simulink model "full_controller_pid"  (R2024a)
settings: Solver=FixedStepAuto  StartTime=0.0  StopTime=50  FixedStep=sample_time  RelTol=1e-3
values from neighbouring files (symbols this model uses):
  dPOSG = [0; 0; 1]    [full_pid_loader.m]
  p_KD = -.01    (= -0.01)    [full_pid_loader.m]
  p_KI = 1    [full_pid_loader.m]
  p_KI_lim = 10*(2*pi/360)    (= 0.174532925199)    [full_pid_loader.m]
  p_KP = 2.7    [full_pid_loader.m]
  phi_KD = 0    [full_pid_loader.m]
  phi_KI = 0    [full_pid_loader.m]
  phi_KI_lim = 2*(2*pi/360)    (= 0.0349065850399)    [full_pid_loader.m]
  phi_KP = 4.5    [full_pid_loader.m]
  phi_max = pi/4    (= 0.785398163397)    [full_pid_loader.m]
  psi_KD = 0    [full_pid_loader.m]
  psi_KI = 0    [full_pid_loader.m]
  psi_KI_lim = 8*(2*pi/360)    (= 0.13962634016)    [full_pid_loader.m]
  psi_KP = 10    [full_pid_loader.m]
  PSIdes = 0    [full_pid_loader.m]
  q_KD = -.01    (= -0.01)    [full_pid_loader.m]
  q_KI = 1    [full_pid_loader.m]
  q_KI_lim = 10*(2*pi/360)    (= 0.174532925199)    [full_pid_loader.m]
  q_KP = 2.7    [full_pid_loader.m]
  r_KD = -.01    (= -0.01)    [full_pid_loader.m]
  r_KI = 1    [full_pid_loader.m]
  r_KI_lim = 10*(2*pi/360)    (= 0.174532925199)    [full_pid_loader.m]
  r_KP = 2.7    [full_pid_loader.m]
  theta_KD = 0    [full_pid_loader.m]
  theta_KI = 0    [full_pid_loader.m]
  theta_KI_lim = 2*(2*pi/360)    (= 0.0349065850399)    [full_pid_loader.m]
  theta_KP = 4.5    [full_pid_loader.m]
  theta_max = pi/4    (= 0.785398163397)    [full_pid_loader.m]
  X_KD = -.35    (= -0.35)    [full_pid_loader.m]
  X_KI = .25    (= 0.25)    [full_pid_loader.m]
  X_KI_lim = 10    [full_pid_loader.m]
  X_KP = .35    (= 0.35)    [full_pid_loader.m]
  Y_KD = -.35    (= -0.35)    [full_pid_loader.m]
  Y_KI = .25    (= 0.25)    [full_pid_loader.m]
  Y_KI_lim = .25    (= 0.25)    [full_pid_loader.m]
  Y_KP = .35    (= 0.35)    [full_pid_loader.m]
undefined symbols (not defined in the file or in its folder): drag_mat, g, J, Jr, m, U_max, U_min
settings Model: Creator=Lorenzo-Desk  LastModifiedBy=Lorenzo-Desk

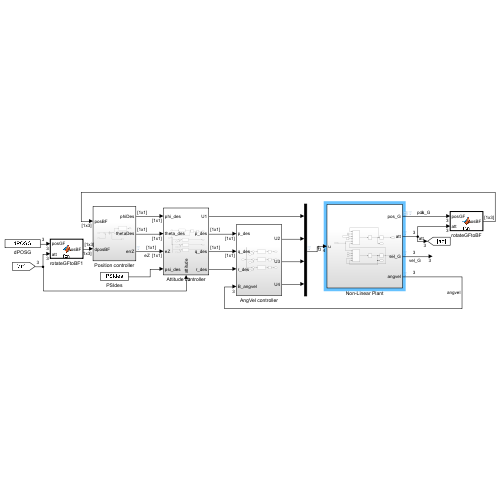
[thumbnail: Simulink's stored preview of the top-level diagram]
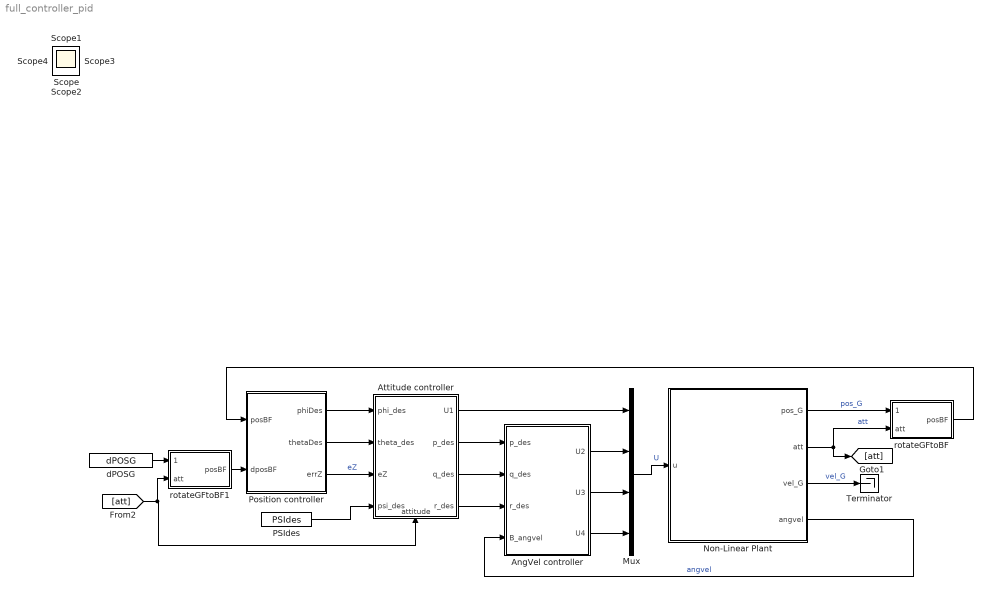
== system full_controller_pid ==
  AngVel controller : Subsystem
  Attitude controller : Subsystem
      settings: PortSchema="{\"entries\":[{\"content\":{\"sides\":[{\"content\":{\"connectorIds\":[\"In1\",\"In2\",\"In3\",\"In4\"]},\"type\":\"ConnectorPlacement.EquallySpacedRectSide\",\"uuid\":\"71281286-38ad-4f2a-91ae-9e6c4e0e30b2\"},{\"content\":{\"connectorIds\":[\"Out1\",\"Out2\",\"Out3\",\"Out4\"],\"side\":\"RIGHT\"},\"type\":\"ConnectorPlacement.EquallySpacedRectSide\",\"uuid\":\"aa649c5f-8758-4d82-8660-affbe0ed2eed\"},{\"content\":{\"side\":\"TOP\"},\"type\":\"ConnectorPlacement.EquallySpacedRectSide\",\"uuid\":\"ccfea5cf-4a16-4d49-8c61-fb0c2c5d9d69\"},{\"content\":{\"connectorIds\":[\"In5\"],\"side\":\"BOTTOM\"},\"type\":\"ConnectorPlacement.EquallySpacedRectSide\",\"uuid\":\"66e9e909-a7d3-4870-b7d3-735590f045d2\"}]},\"type\":\"ConnectorPlacement.EquallySpacedConnector\",\"uuid\":\"1ea574e8-8b7c-489a-8841-cd1e9d9d608b\"}],\"packageUris\":[\"http://schema.mathworks.com/mf0/Connector/R2020b\"],\"version\":\"1.0\"}"
  Mux : Mux
  Non-Linear Plant : Subsystem
  PSIdes : Constant  Value=PSIdes
  Position controller : Subsystem
  Terminator : Terminator
  dPOSG : Constant  Value=dPOSG
  rotateGFtoBF : MATLAB Function  TreatAsAtomicUnit=on
  rotateGFtoBF1 : MATLAB Function  TreatAsAtomicUnit=on
  Scope{,1..4} (5 alike) : Scope
  wires:
  Non-Linear Plant/1(pos_G) -> rotateGFtoBF/1(posGF)  "pos_G"
  Attitude controller/2(p_des) -> AngVel controller/1(p_des)
  PSIdes/1 -> Attitude controller/4(psi_des)
  Attitude controller/3(q_des) -> AngVel controller/2(q_des)
  Attitude controller/4(r_des) -> AngVel controller/3(r_des)
  Attitude controller/1(U1) -> Mux/1
  AngVel controller/1(U2) -> Mux/2
  AngVel controller/2(U3) -> Mux/3
  AngVel controller/3(U4) -> Mux/4
  Non-Linear Plant/2(att) -> [att], rotateGFtoBF/2(att)  "att"
  Non-Linear Plant/4(angvel) -> AngVel controller/4(B_angvel)  "angvel"
  Non-Linear Plant/3(vel_G) -> Terminator/1  "vel_G"
  Position controller/3(errZ) -> Attitude controller/3(eZ)  "eZ"
  Position controller/1(phiDes) -> Attitude controller/1(phi_des)
  Position controller/2(thetaDes) -> Attitude controller/2(theta_des)
  Mux/1 -> Non-Linear Plant/1(u)  "U"
  rotateGFtoBF/1(posBF) -> Position controller/1(posBF)
  rotateGFtoBF1/1(posBF) -> Position controller/2(dposBF)
  dPOSG/1 -> rotateGFtoBF1/1(posGF)
  [att] -> Attitude controller/5(attitude), rotateGFtoBF1/2(att)

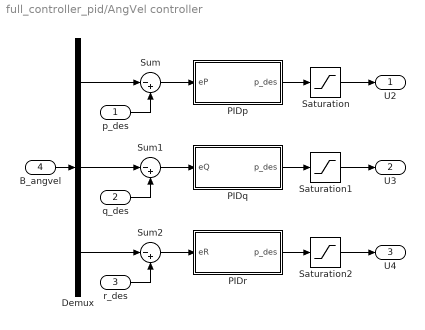
== system full_controller_pid/AngVel controller ==
  p_des : Inport
  q_des : Inport  Port=2
  r_des : Inport  Port=3
  B_angvel : Inport  Port=4
  Demux : Demux  Outputs=3
  PIDp : Subsystem
  PIDq : Subsystem
  PIDr : Subsystem
  Saturation : Saturate  UpperLimit=U_max(2)  LowerLimit=U_min(2)
  Saturation1 : Saturate  UpperLimit=U_max(3)  LowerLimit=U_min(3)
  Saturation2 : Saturate  UpperLimit=U_max(4)  LowerLimit=U_min(4)
  Sum : Sum  Inputs=|-+
  Sum1 : Sum  Inputs=|-+
  Sum2 : Sum  Inputs=|-+
  U2 : Outport
  U3 : Outport  Port=2
  U4 : Outport  Port=3
  wires:
  PIDp/1(p_des) -> Saturation/1
  PIDq/1(p_des) -> Saturation1/1
  PIDr/1(p_des) -> Saturation2/1
  Sum/1 -> PIDp/1(eP)
  Sum1/1 -> PIDq/1(eQ)
  Sum2/1 -> PIDr/1(eR)
  p_des/1 -> Sum/2
  q_des/1 -> Sum1/2
  r_des/1 -> Sum2/2
  B_angvel/1 -> Demux/1
  Demux/1 -> Sum/1
  Demux/2 -> Sum1/1
  Demux/3 -> Sum2/1
  Saturation/1 -> U2/1
  Saturation1/1 -> U3/1
  Saturation2/1 -> U4/1

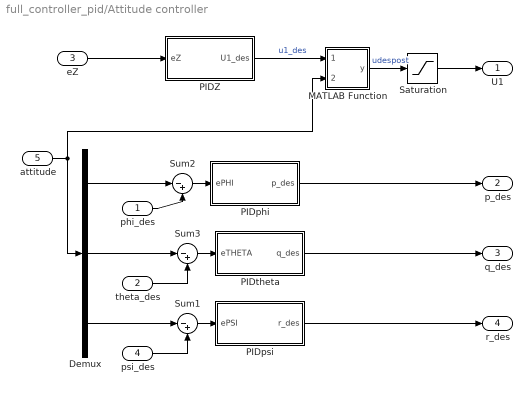
== system full_controller_pid/Attitude controller ==
  phi_des : Inport
  theta_des : Inport  Port=2
  eZ : Inport  Port=3
  psi_des : Inport  Port=4
  attitude : Inport  Port=5
  Demux : Demux  Outputs=3
  MATLAB Function : MATLAB Function  TreatAsAtomicUnit=on
  PIDZ : Subsystem
  PIDphi : Subsystem
  PIDpsi : Subsystem
  PIDtheta : Subsystem
  Saturation : Saturate  UpperLimit=U_max(1)  LowerLimit=U_min(1)
  Sum1 : Sum  Inputs=|-+
  Sum2 : Sum  Inputs=|-+
  Sum3 : Sum  Inputs=|-+
  U1 : Outport
  p_des : Outport  Port=2
  q_des : Outport  Port=3
  r_des : Outport  Port=4
  wires:
  PIDZ/1(U1_des) -> MATLAB Function/1(pidOut)  "u1_des"
  attitude/1 -> Demux/1, MATLAB Function/2(angles)
  eZ/1 -> PIDZ/1(eZ)
  PIDphi/1(p_des) -> p_des/1
  PIDtheta/1(q_des) -> q_des/1
  Sum2/1 -> PIDphi/1(ePHI)
  phi_des/1 -> Sum2/2
  Demux/1 -> Sum2/1
  Sum3/1 -> PIDtheta/1(eTHETA)
  theta_des/1 -> Sum3/2
  Demux/2 -> Sum3/1
  Demux/3 -> Sum1/1
  psi_des/1 -> Sum1/2
  Sum1/1 -> PIDpsi/1(ePSI)
  PIDpsi/1(r_des) -> r_des/1
  MATLAB Function/1(y) -> Saturation/1  "udespost"
  Saturation/1 -> U1/1

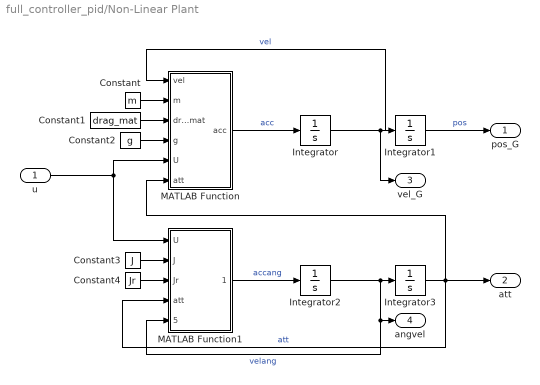
== system full_controller_pid/Non-Linear Plant ==
  u : Inport  PortDimensions=4
  Constant : Constant  Value=m
  Constant1 : Constant  Value=drag_mat
  Constant2 : Constant  Value=g
  Constant3 : Constant  Value=J
  Constant4 : Constant  Value=Jr
  Integrator{,1..3} (4 alike) : Integrator
  MATLAB Function : MATLAB Function  TreatAsAtomicUnit=on
  MATLAB Function1 : MATLAB Function  TreatAsAtomicUnit=on
  pos_G : Outport  PortDimensions=3
  att : Outport  Port=2  PortDimensions=3
  vel_G : Outport  Port=3
  angvel : Outport  Port=4
  wires:
  u/1 -> MATLAB Function1/1(U), MATLAB Function/5(U)
  Integrator2/1 -> angvel/1, MATLAB Function1/5(velang), Integrator3/1  "velang"
  Constant4/1 -> MATLAB Function1/3(Jr)
  MATLAB Function/1(acc) -> Integrator/1  "acc"
  Integrator/1 -> vel_G/1, Integrator1/1, MATLAB Function/1(vel)  "vel"
  Constant/1 -> MATLAB Function/2(m)
  Integrator3/1 -> MATLAB Function1/4(att), att/1, MATLAB Function/6(att)  "att"
  MATLAB Function1/1(accang) -> Integrator2/1  "accang"
  Integrator1/1 -> pos_G/1  "pos"
  Constant1/1 -> MATLAB Function/3(drag_mat)
  Constant2/1 -> MATLAB Function/4(g)
  Constant3/1 -> MATLAB Function1/2(J)

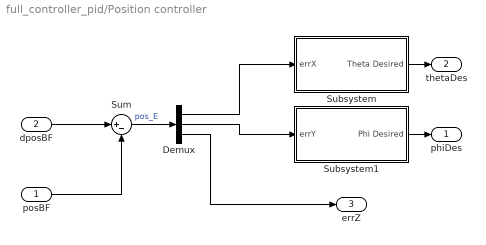
== system full_controller_pid/Position controller ==
  posBF : Inport
  dposBF : Inport  Port=2
  Demux : Demux  Outputs=3
  Subsystem : Subsystem
  Subsystem1 : Subsystem
  Sum : Sum  Inputs=|+-
  phiDes : Outport
  thetaDes : Outport  Port=2
  errZ : Outport  Port=3
  wires:
  posBF/1 -> Sum/2
  Sum/1 -> Demux/1  "pos_E"
  dposBF/1 -> Sum/1
  Demux/1 -> Subsystem/1(errX)
  Demux/2 -> Subsystem1/1(errY)
  Demux/3 -> errZ/1
  Subsystem/1(Theta Desired) -> thetaDes/1
  Subsystem1/1(Phi Desired) -> phiDes/1

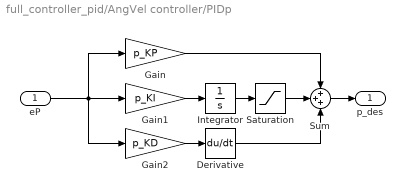
== system full_controller_pid/AngVel controller/PIDp ==
  eP : Inport
  Derivative : Derivative
  Gain : Gain  Gain=p_KP
  Gain1 : Gain  Gain=p_KI
  Gain2 : Gain  Gain=p_KD
  Integrator : Integrator
  Saturation : Saturate  UpperLimit=p_KI_lim  LowerLimit=-p_KI_lim
  Sum : Sum  Inputs=+++
  p_des : Outport
  wires:
  Integrator/1 -> Saturation/1
  Derivative/1 -> Sum/3
  Gain/1 -> Sum/1
  Sum/1 -> p_des/1
  eP/1 -> Gain/1, Gain1/1, Gain2/1
  Gain1/1 -> Integrator/1
  Gain2/1 -> Derivative/1
  Saturation/1 -> Sum/2

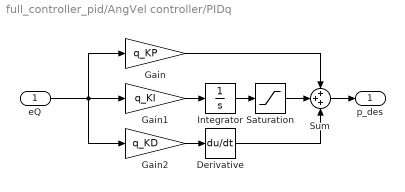
== system full_controller_pid/AngVel controller/PIDq ==
  eQ : Inport
  Derivative : Derivative
  Gain : Gain  Gain=q_KP
  Gain1 : Gain  Gain=q_KI
  Gain2 : Gain  Gain=q_KD
  Integrator : Integrator
  Saturation : Saturate  UpperLimit=q_KI_lim  LowerLimit=-q_KI_lim
  Sum : Sum  Inputs=+++
  p_des : Outport
  wires:
  Gain2/1 -> Derivative/1
  Integrator/1 -> Saturation/1
  Gain/1 -> Sum/1
  Sum/1 -> p_des/1
  Gain1/1 -> Integrator/1
  Derivative/1 -> Sum/3
  eQ/1 -> Gain/1, Gain1/1, Gain2/1
  Saturation/1 -> Sum/2

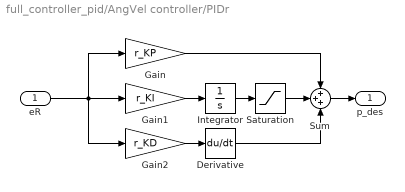
== system full_controller_pid/AngVel controller/PIDr ==
  eR : Inport
  Derivative : Derivative
  Gain : Gain  Gain=r_KP
  Gain1 : Gain  Gain=r_KI
  Gain2 : Gain  Gain=r_KD
  Integrator : Integrator
  Saturation : Saturate  UpperLimit=r_KI_lim  LowerLimit=-r_KI_lim
  Sum : Sum  Inputs=+++
  p_des : Outport
  wires:
  Gain2/1 -> Derivative/1
  Integrator/1 -> Saturation/1
  Gain/1 -> Sum/1
  Sum/1 -> p_des/1
  Gain1/1 -> Integrator/1
  Derivative/1 -> Sum/3
  eR/1 -> Gain/1, Gain1/1, Gain2/1
  Saturation/1 -> Sum/2

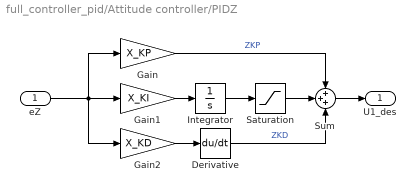
== system full_controller_pid/Attitude controller/PIDZ ==
  eZ : Inport
  Derivative : Derivative
  Gain : Gain  Gain=X_KP
  Gain1 : Gain  Gain=X_KI
  Gain2 : Gain  Gain=X_KD
  Integrator : Integrator
  Saturation : Saturate  UpperLimit=X_KI_lim  LowerLimit=-X_KI_lim
  Sum : Sum  Inputs=+++
  U1_des : Outport
  wires:
  Integrator/1 -> Saturation/1
  Derivative/1 -> Sum/3  "ZKD"
  Gain/1 -> Sum/1  "ZKP"
  Sum/1 -> U1_des/1
  eZ/1 -> Gain2/1, Gain1/1, Gain/1
  Gain1/1 -> Integrator/1
  Gain2/1 -> Derivative/1
  Saturation/1 -> Sum/2

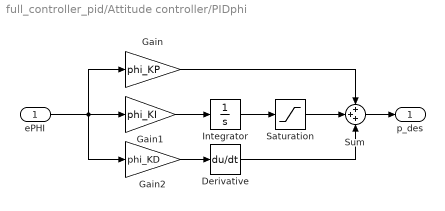
== system full_controller_pid/Attitude controller/PIDphi ==
  ePHI : Inport
  Derivative : Derivative
  Gain : Gain  Gain=phi_KP
  Gain1 : Gain  Gain=phi_KI
  Gain2 : Gain  Gain=phi_KD
  Integrator : Integrator
  Saturation : Saturate  UpperLimit=phi_KI_lim  LowerLimit=-phi_KI_lim
  Sum : Sum  Inputs=+++
  p_des : Outport
  wires:
  ePHI/1 -> Gain2/1, Gain1/1, Gain/1
  Sum/1 -> p_des/1
  Gain/1 -> Sum/1
  Derivative/1 -> Sum/3
  Integrator/1 -> Saturation/1
  Gain1/1 -> Integrator/1
  Gain2/1 -> Derivative/1
  Saturation/1 -> Sum/2

== system full_controller_pid/Attitude controller/PIDpsi ==
  ePSI : Inport
  Derivative : Derivative
  Gain : Gain  Gain=psi_KP
  Gain1 : Gain  Gain=psi_KI
  Gain2 : Gain  Gain=psi_KD
  Integrator : Integrator
  Saturation : Saturate  UpperLimit=psi_KI_lim  LowerLimit=-psi_KI_lim
  Sum : Sum  Inputs=+++
  r_des : Outport
  wires:
  ePSI/1 -> Gain2/1, Gain1/1, Gain/1
  Sum/1 -> r_des/1
  Gain/1 -> Sum/1
  Derivative/1 -> Sum/3
  Integrator/1 -> Saturation/1
  Gain1/1 -> Integrator/1
  Gain2/1 -> Derivative/1
  Saturation/1 -> Sum/2

== system full_controller_pid/Attitude controller/PIDtheta ==
  eTHETA : Inport
  Derivative : Derivative
  Gain : Gain  Gain=theta_KP
  Gain1 : Gain  Gain=theta_KI
  Gain2 : Gain  Gain=theta_KD
  Integrator : Integrator
  Saturation : Saturate  UpperLimit=theta_KI_lim  LowerLimit=-theta_KI_lim
  Sum : Sum  Inputs=+++
  q_des : Outport
  wires:
  Integrator/1 -> Saturation/1
  Derivative/1 -> Sum/3
  Gain/1 -> Sum/1
  Sum/1 -> q_des/1
  eTHETA/1 -> Gain/1, Gain1/1, Gain2/1
  Gain1/1 -> Integrator/1
  Gain2/1 -> Derivative/1
  Saturation/1 -> Sum/2

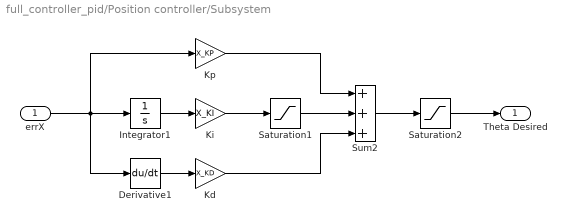
== system full_controller_pid/Position controller/Subsystem ==
  errX : Inport
  Derivative1 : Derivative
  Integrator1 : Integrator
  Kd : Gain  Gain=X_KD
  Ki : Gain  Gain=X_KI
  Kp : Gain  Gain=X_KP
  Saturation1 : Saturate  UpperLimit=X_KI_lim  LowerLimit=-X_KI_lim
  Saturation2 : Saturate  UpperLimit=theta_max  LowerLimit=-theta_max
  Sum2 : Sum  Inputs=+++
  Theta Desired : Outport
  wires:
  Derivative1/1 -> Kd/1
  Kp/1 -> Sum2/1
  Kd/1 -> Sum2/3
  Saturation2/1 -> Theta Desired/1
  Sum2/1 -> Saturation2/1
  Integrator1/1 -> Ki/1
  errX/1 -> Derivative1/1, Integrator1/1, Kp/1
  Saturation1/1 -> Sum2/2
  Ki/1 -> Saturation1/1

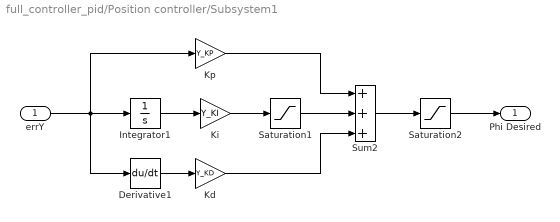
== system full_controller_pid/Position controller/Subsystem1 ==
  errY : Inport
  Derivative1 : Derivative
  Integrator1 : Integrator
  Kd : Gain  Gain=Y_KD
  Ki : Gain  Gain=Y_KI
  Kp : Gain  Gain=Y_KP
  Saturation1 : Saturate  UpperLimit=Y_KI_lim  LowerLimit=-Y_KI_lim
  Saturation2 : Saturate  UpperLimit=phi_max  LowerLimit=-phi_max
  Sum2 : Sum  Inputs=+++
  Phi Desired : Outport
  wires:
  Ki/1 -> Saturation1/1
  Saturation1/1 -> Sum2/2
  errY/1 -> Kp/1, Integrator1/1, Derivative1/1
  Integrator1/1 -> Ki/1
  Sum2/1 -> Saturation2/1
  Saturation2/1 -> Phi Desired/1
  Kd/1 -> Sum2/3
  Kp/1 -> Sum2/1
  Derivative1/1 -> Kd/1

== matlab function full_controller_pid/Non-Linear Plant/MATLAB Function ==
  data: vel input; m input; drag_mat input; g input; U input; att input; acc output
function acc = fcn(vel, m, drag_mat, g, U, att)
u = vel(1); v = vel(2); w = vel(3);
phi = att(1); theta = att(2); psi = att(3);
kdx = drag_mat(1,1); kdy = drag_mat(2,2); kdz = drag_mat(3,3);
acc = zeros(3,1);
acc(1) = (-(cos(phi)*sin(theta)*cos(psi) + sin(phi)*sin(psi))*U(1) - kdx*u)/m;
acc(2) = (-(cos(phi)*sin(theta)*sin(psi) - sin(phi) * cos(psi))*U(1) - kdy*v)/m;
acc(3) = (-(cos(phi)*cos(theta))*U(1) - kdz * w)/m + g;

== matlab function full_controller_pid/Attitude controller/MATLAB Function ==
  data: pidOut input; y output; angles input
function y = fcn(pidOut, angles)
phi = angles(1);
theta = angles(2);
y = 1/(cos(phi)*cos(theta))*pidOut;

== matlab function full_controller_pid/Non-Linear Plant/MATLAB Function1 ==
  data: U input; accang output; J input; Jr input; att input; velang input
function accang = fcn(U, J, Jr, att, velang)
Jx = J(1); Jy = J(2); Jz = J(3);
phi = att(1); theta = att(2); psi = att(3);
B_phi_dot = velang(1); B_theta_dot = velang(2); B_psi_dot = velang(3);

accang = zeros(3,1);
accang(1) = (Jy-Jz/Jx)*B_theta_dot*B_psi_dot-Jr/Jx*B_theta_dot*U(1)+U(2)/Jx;
accang(2) = (Jz-Jx/Jy)*B_phi_dot*B_psi_dot+Jr/Jy*B_phi_dot*U(1)+U(3)/Jy;
accang(3) = (Jx-Jy/Jz)*B_phi_dot*B_theta_dot+U(4)/Jz;

%phi_dot = velang(1); theta_dot = velang(2); psi_dot = velang(3);
%y(1) = (Jy-Jz/Jx)*theta_dot*psi_dot-Jr/Jx*theta_dot*u(1)+u(2)/Jx;
%y(2) = (Jz-Jx/Jy)*phi_dot*psi_dot+Jr/Jy*phi_dot*u(1)+u(3)/Jy;
%y(3) = (Jx-Jy/Jz)*phi_dot*theta_dot+u(4)/Jz;

== matlab function full_controller_pid/rotateGFtoBF1 ==
  data: posGF input; posBF output; att input
function posBF = fcn(posGF, att)
phi = att(1); theta = att(2); psi = att(3);
R_roll = [...
      1, 0, 0;...
      0, cos(phi), -sin(phi);...
      0, sin(phi), cos(phi)];
R_pitch = [...
      cos(theta), 0, sin(theta);...
      0, 1, 0;...
      -sin(theta), 0, cos(theta)];
R_yaw = [...
      cos(psi), -sin(psi), 0;...
      sin(psi), cos(psi), 0;...
      0, 0, 1];  
  
R = R_yaw*R_pitch*R_roll;
posBF = posGF'*R;

== matlab function full_controller_pid/rotateGFtoBF ==
  data: posGF input; posBF output; att input
function posBF = fcn(posGF, att)
phi = att(1); theta = att(2); psi = att(3);
R_roll = [...
      1, 0, 0;...
      0, cos(phi), -sin(phi);...
      0, sin(phi), cos(phi)];
R_pitch = [...
      cos(theta), 0, sin(theta);...
      0, 1, 0;...
      -sin(theta), 0, cos(theta)];
R_yaw = [...
      cos(psi), -sin(psi), 0;...
      sin(psi), cos(psi), 0;...
      0, 0, 1];  
  
R = R_yaw*R_pitch*R_roll;
posBF = posGF'*R;
